simulink model "c00020M_harness"  (R2018a)
settings: Solver=ode3  StartTime=0.0  StopTime=10.0  RelTol=1e-3  EnableMultiTasking=on
undefined symbols (not defined in the file): b, DiscIntNeverNeededParam, J, K, L, PosMinimaW4, R, sigbuilder_block
(part 1 of 41)
settings Model: Creator=aarrieta  LastModifiedBy=umarkiegi
settings DataIOCC: LimitDataPoints=on  SaveFormat=Array
settings OptimizationCC: LifeSpan=inf
settings DebuggingCC: UnderspecifiedInitializationDetection=Classic  MergeDetectMultiDrivingBlocksExec=none  SolverPrmCheckMsg=warning  StateNameClashWarn=warning  SFUnexpectedBacktrackingDiag=warning  SFNoUnconditionalDefaultTransitionDiag=warning  SFExecutionAtInitializationDiag=none
settings HardwareCC: ProdBitPerPointer=32  ProdBitPerSizeT=32  ProdBitPerPtrDiffT=32  ProdLargestAtomicFloat=None  ProdIntDivRoundTo=Undefined  ProdEndianess=Unspecified  ProdWordSize=32  ProdHWDeviceType=32-bit Generic
settings ModelReferenceCC: PropagateSignalLabelsOutOfModel=off
settings CodeAppCC: StateflowObjectComments=on
settings GRTTargetCC: TargetLangStandard=C89/C90 (ANSI)  GeneratePreprocessorConditionals=Disable all
settings ConfigComp: CovMetricSettings=dw  CovHtmlReporting=on  CovSaveCumulativeToWorkspaceVar=on  CovSaveSingleToWorkspaceVar=on  CovExternalEMLEnable=off  DVMaxTestCaseSteps=20  DVTestSuiteOptimization=CombinedObjectives (Nonlinear Extended)  DVDetectFloatOverflow=off

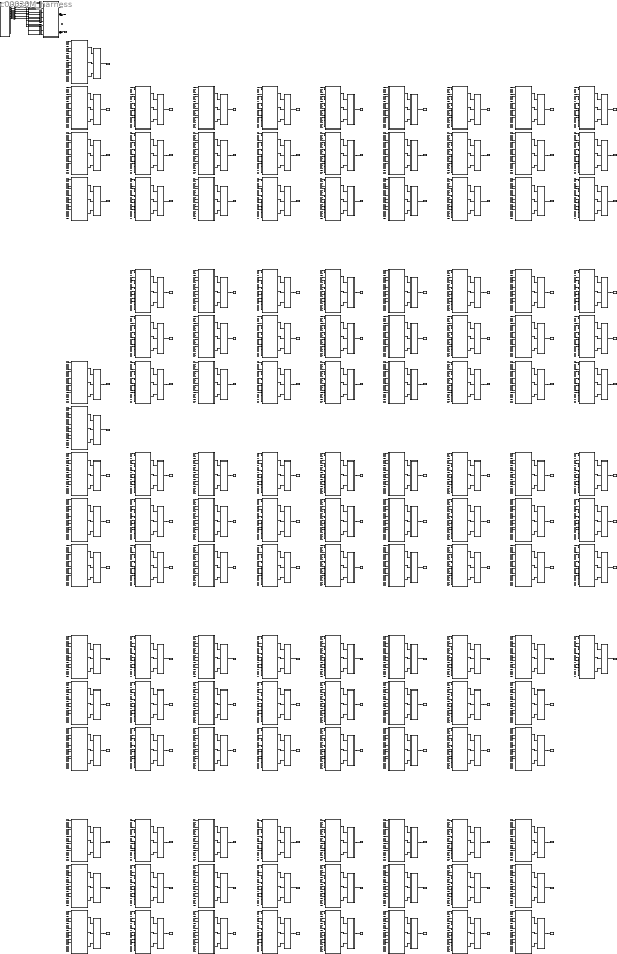
== system c00020M_harness ==
  CPSUT : Subsystem
  Eval : Subsystem
  Eval1 : Subsystem
  Eval10 : Subsystem
  Eval101 : Subsystem
  Eval102 : Subsystem
  Eval103 : Subsystem
  Eval105 : Subsystem
  Eval106 : Subsystem
  Eval107 : Subsystem
  Eval109 : Subsystem
  Eval11 : Subsystem
  Eval110 : Subsystem
  Eval111 : Subsystem
  Eval113 : Subsystem
  Eval114 : Subsystem
  Eval115 : Subsystem
  Eval117 : Subsystem
  Eval118 : Subsystem
  Eval119 : Subsystem
  Eval121 : Subsystem
  Eval122 : Subsystem
  Eval123 : Subsystem
  Eval125 : Subsystem
  Eval126 : Subsystem
  Eval127 : Subsystem
  Eval129 : Subsystem
  Eval13 : Subsystem
  Eval130 : Subsystem
  Eval131 : Subsystem
  Eval133 : Subsystem
  Eval134 : Subsystem
  Eval135 : Subsystem
  Eval137 : Subsystem
  Eval138 : Subsystem
  Eval139 : Subsystem
  Eval14 : Subsystem
  Eval141 : Subsystem
  Eval142 : Subsystem
  Eval143 : Subsystem
  Eval145 : Subsystem
  Eval146 : Subsystem
  Eval147 : Subsystem
  Eval149 : Subsystem
  Eval15 : Subsystem
  Eval150 : Subsystem
  Eval151 : Subsystem
  Eval153 : Subsystem
  Eval154 : Subsystem
  Eval155 : Subsystem
  Eval157 : Subsystem
  Eval158 : Subsystem
  Eval159 : Subsystem
  Eval161 : Subsystem
  Eval162 : Subsystem
  Eval163 : Subsystem
  Eval165 : Subsystem
  Eval166 : Subsystem
  Eval167 : Subsystem
  Eval169 : Subsystem
  Eval17 : Subsystem
  Eval170 : Subsystem
  Eval171 : Subsystem
  Eval173 : Subsystem
  Eval18 : Subsystem
  Eval19 : Subsystem
  Eval2 : Subsystem
  Eval21 : Subsystem
  Eval22 : Subsystem
  Eval23 : Subsystem
  Eval25 : Subsystem
  Eval26 : Subsystem
  Eval27 : Subsystem
  Eval29 : Subsystem
  Eval3 : Subsystem
  Eval30 : Subsystem
  Eval31 : Subsystem
  Eval33 : Subsystem
  Eval34 : Subsystem
  Eval35 : Subsystem
  Eval37 : Subsystem
  Eval38 : Subsystem
  Eval39 : Subsystem
  Eval41 : Subsystem
  Eval42 : Subsystem
  Eval43 : Subsystem
  Eval45 : Subsystem
  Eval46 : Subsystem
  Eval47 : Subsystem
  Eval49 : Subsystem
  Eval50 : Subsystem
  Eval51 : Subsystem
  Eval53 : Subsystem
  Eval54 : Subsystem
  Eval55 : Subsystem
  Eval57 : Subsystem
  Eval58 : Subsystem
  Eval59 : Subsystem
  Eval61 : Subsystem
  Eval62 : Subsystem
  Eval63 : Subsystem
  Eval65 : Subsystem
  Eval66 : Subsystem
  Eval67 : Subsystem
  Eval69 : Subsystem
  Eval7 : Subsystem
  Eval70 : Subsystem
  Eval71 : Subsystem
  Eval73 : Subsystem
  Eval74 : Subsystem
  Eval75 : Subsystem
  Eval77 : Subsystem
  Eval78 : Subsystem
  Eval79 : Subsystem
  Eval8 : Subsystem
  Eval81 : Subsystem
  Eval82 : Subsystem
  Eval83 : Subsystem
  Eval85 : Subsystem
  Eval86 : Subsystem
  Eval87 : Subsystem
  Eval89 : Subsystem
  Eval9 : Subsystem
  Eval90 : Subsystem
  Eval91 : Subsystem
  Eval93 : Subsystem
  Eval94 : Subsystem
  Eval95 : Subsystem
  Eval97 : Subsystem
  Eval98 : Subsystem
  Eval99 : Subsystem
  Inputs : Subsystem  Tag=STV Subsys  LoadFcn=sigbuilder_block('load');  StartFcn=sigbuilder_block('start');  StopFcn=sigbuilder_block('stop');  ClipboardFcn=sigbuilder_block('clipboard');  mask(Sigbuilder block){tuvar=[0:10]}
      mask init:
      | if ~strcmp(get_param(bdroot(gcb),'SimulationStatus'),'stopped'),tuvar = sigbuilder_block('maskInit'); end
      settings: CopyFcn=sigbuilder_block('copy');  DeleteFcn=sigbuilder_block('delete');  ModelCloseFcn=sigbuilder_block('modelClose');  PreSaveFcn=sigbuilder_block('preSave');  PauseFcn=sigbuilder_block('pause');  ContinueFcn=sigbuilder_block('continue');  NameChangeFcn=sigbuilder_block('namechange');  OpenFcn=sigbuilder_block('open');  CloseFcn=sigbuilder_block('close');
      mask Display: plot(0, 0, 100, 100,[2, 2, 32, 32, 2], [68, 8, 8, 68, 68],[32, 2], [38, 38], [32, 19, 2],[53, 60, 44], [32, 17, 17, 2],[16, 16, 31, 31]);txt = getActiveGroup(gcbh);text(2, 100, txt,'verticalAlignment', 'top');
  M001 : Subsystem
  M002 : Subsystem
  M003 : Subsystem
  M004 : Subsystem
  M008 : Subsystem
  M009 : Subsystem
  M010 : Subsystem
  M011 : Subsystem
  M012 : Subsystem
  M014 : Subsystem
  M015 : Subsystem
  M016 : Subsystem
  M018 : Subsystem
  M019 : Subsystem
  M020 : Subsystem
  M022 : Subsystem
  M023 : Subsystem
  M024 : Subsystem
  M026 : Subsystem
  M027 : Subsystem
  M028 : Subsystem
  M030 : Subsystem
  M031 : Subsystem
  M032 : Subsystem
  M034 : Subsystem
  M035 : Subsystem
  M036 : Subsystem
  M038 : Subsystem
  M039 : Subsystem
  M040 : Subsystem
  M042 : Subsystem
  M043 : Subsystem
  M044 : Subsystem
  M046 : Subsystem
  M047 : Subsystem
  M048 : Subsystem
  M050 : Subsystem
  M051 : Subsystem
  M052 : Subsystem
  M054 : Subsystem
  M055 : Subsystem
  M056 : Subsystem
  M058 : Subsystem
  M059 : Subsystem
  M060 : Subsystem
  M062 : Subsystem
  M063 : Subsystem
  M064 : Subsystem
  M066 : Subsystem
  M067 : Subsystem
  M068 : Subsystem
  M070 : Subsystem
  M071 : Subsystem
  M072 : Subsystem
  M074 : Subsystem
  M075 : Subsystem
  M076 : Subsystem
  M078 : Subsystem
  M079 : Subsystem
  M080 : Subsystem
  M082 : Subsystem
  M083 : Subsystem
  M084 : Subsystem
  M086 : Subsystem
  M087 : Subsystem
  M088 : Subsystem
  M090 : Subsystem
  M091 : Subsystem
  M092 : Subsystem
  M094 : Subsystem
  M095 : Subsystem
  M096 : Subsystem
  M098 : Subsystem
  M099 : Subsystem
  M100 : Subsystem
  M102 : Subsystem
  M103 : Subsystem
  M104 : Subsystem
  M106 : Subsystem
  M107 : Subsystem
  M108 : Subsystem
  M110 : Subsystem
  M111 : Subsystem
  M112 : Subsystem
  M114 : Subsystem
  M115 : Subsystem
  M116 : Subsystem
  M118 : Subsystem
  M119 : Subsystem
  M120 : Subsystem
  M122 : Subsystem
  M123 : Subsystem
  M124 : Subsystem
  M126 : Subsystem
  M127 : Subsystem
  M128 : Subsystem
  M130 : Subsystem
  M131 : Subsystem
  M132 : Subsystem
  M134 : Subsystem
  M135 : Subsystem
  M136 : Subsystem
  M138 : Subsystem
  M139 : Subsystem
  M140 : Subsystem
  M142 : Subsystem
  M143 : Subsystem
  M144 : Subsystem
  M146 : Subsystem
  M147 : Subsystem
  M148 : Subsystem
  M150 : Subsystem
  M151 : Subsystem
  M152 : Subsystem
  M154 : Subsystem
  M155 : Subsystem
  M156 : Subsystem
  M158 : Subsystem
  M159 : Subsystem
  M160 : Subsystem
  M162 : Subsystem
  M163 : Subsystem
  M164 : Subsystem
  M166 : Subsystem
  M167 : Subsystem
  M168 : Subsystem
  M170 : Subsystem
  M171 : Subsystem
  M172 : Subsystem
  M174 : Subsystem
  To Workspace : ToWorkspace  VariableName=mutant001  SampleTime=-1
  To Workspace1 : ToWorkspace  VariableName=mutant002  SampleTime=-1
  To Workspace10 : ToWorkspace  VariableName=mutant011  SampleTime=-1
  To Workspace101 : ToWorkspace  VariableName=mutant102  SampleTime=-1
  To Workspace102 : ToWorkspace  VariableName=mutant103  SampleTime=-1
  To Workspace103 : ToWorkspace  VariableName=mutant104  SampleTime=-1
  To Workspace105 : ToWorkspace  VariableName=mutant106  SampleTime=-1
  To Workspace106 : ToWorkspace  VariableName=mutant107  SampleTime=-1
  To Workspace107 : ToWorkspace  VariableName=mutant108  SampleTime=-1
  To Workspace109 : ToWorkspace  VariableName=mutant110  SampleTime=-1
  To Workspace11 : ToWorkspace  VariableName=mutant012  SampleTime=-1
  To Workspace110 : ToWorkspace  VariableName=mutant111  SampleTime=-1
  To Workspace111 : ToWorkspace  VariableName=mutant112  SampleTime=-1
  To Workspace113 : ToWorkspace  VariableName=mutant114  SampleTime=-1
  To Workspace114 : ToWorkspace  VariableName=mutant115  SampleTime=-1
  To Workspace115 : ToWorkspace  VariableName=mutant116  SampleTime=-1
  To Workspace117 : ToWorkspace  VariableName=mutant118  SampleTime=-1
  To Workspace118 : ToWorkspace  VariableName=mutant119  SampleTime=-1
  To Workspace119 : ToWorkspace  VariableName=mutant120  SampleTime=-1
  To Workspace121 : ToWorkspace  VariableName=mutant122  SampleTime=-1
  To Workspace122 : ToWorkspace  VariableName=mutant123  SampleTime=-1
  To Workspace123 : ToWorkspace  VariableName=mutant124  SampleTime=-1
  To Workspace125 : ToWorkspace  VariableName=mutant126  SampleTime=-1
  To Workspace126 : ToWorkspace  VariableName=mutant127  SampleTime=-1
  To Workspace127 : ToWorkspace  VariableName=mutant128  SampleTime=-1
  To Workspace129 : ToWorkspace  VariableName=mutant130  SampleTime=-1
  To Workspace13 : ToWorkspace  VariableName=mutant014  SampleTime=-1
  To Workspace130 : ToWorkspace  VariableName=mutant131  SampleTime=-1
  To Workspace131 : ToWorkspace  VariableName=mutant132  SampleTime=-1
  To Workspace133 : ToWorkspace  VariableName=mutant134  SampleTime=-1
  To Workspace134 : ToWorkspace  VariableName=mutant135  SampleTime=-1
  To Workspace135 : ToWorkspace  VariableName=mutant136  SampleTime=-1
  To Workspace137 : ToWorkspace  VariableName=mutant138  SampleTime=-1
  To Workspace138 : ToWorkspace  VariableName=mutant139  SampleTime=-1
  To Workspace139 : ToWorkspace  VariableName=mutant140  SampleTime=-1
  To Workspace14 : ToWorkspace  VariableName=mutant015  SampleTime=-1
  To Workspace141 : ToWorkspace  VariableName=mutant142  SampleTime=-1
  To Workspace142 : ToWorkspace  VariableName=mutant143  SampleTime=-1
  To Workspace143 : ToWorkspace  VariableName=mutant144  SampleTime=-1
  To Workspace145 : ToWorkspace  VariableName=mutant146  SampleTime=-1
  To Workspace146 : ToWorkspace  VariableName=mutant147  SampleTime=-1
  To Workspace147 : ToWorkspace  VariableName=mutant148  SampleTime=-1
  To Workspace149 : ToWorkspace  VariableName=mutant150  SampleTime=-1
  To Workspace15 : ToWorkspace  VariableName=mutant016  SampleTime=-1
  To Workspace150 : ToWorkspace  VariableName=mutant151  SampleTime=-1
  To Workspace151 : ToWorkspace  VariableName=mutant152  SampleTime=-1
  To Workspace153 : ToWorkspace  VariableName=mutant154  SampleTime=-1
  To Workspace154 : ToWorkspace  VariableName=mutant155  SampleTime=-1
  To Workspace155 : ToWorkspace  VariableName=mutant156  SampleTime=-1
  To Workspace157 : ToWorkspace  VariableName=mutant158  SampleTime=-1
  To Workspace158 : ToWorkspace  VariableName=mutant159  SampleTime=-1
  To Workspace159 : ToWorkspace  VariableName=mutant160  SampleTime=-1
  To Workspace161 : ToWorkspace  VariableName=mutant162  SampleTime=-1
  To Workspace162 : ToWorkspace  VariableName=mutant163  SampleTime=-1
  To Workspace163 : ToWorkspace  VariableName=mutant164  SampleTime=-1
  To Workspace165 : ToWorkspace  VariableName=mutant166  SampleTime=-1
  To Workspace166 : ToWorkspace  VariableName=mutant167  SampleTime=-1
  To Workspace167 : ToWorkspace  VariableName=mutant168  SampleTime=-1
  To Workspace169 : ToWorkspace  VariableName=mutant170  SampleTime=-1
  To Workspace17 : ToWorkspace  VariableName=mutant018  SampleTime=-1
  To Workspace170 : ToWorkspace  VariableName=mutant171  SampleTime=-1
  To Workspace171 : ToWorkspace  VariableName=mutant172  SampleTime=-1
  To Workspace173 : ToWorkspace  VariableName=mutant174  SampleTime=-1
  To Workspace18 : ToWorkspace  VariableName=mutant019  SampleTime=-1
  To Workspace19 : ToWorkspace  VariableName=mutant020  SampleTime=-1
  To Workspace2 : ToWorkspace  VariableName=mutant003  SampleTime=-1
  To Workspace21 : ToWorkspace  VariableName=mutant022  SampleTime=-1
  To Workspace22 : ToWorkspace  VariableName=mutant023  SampleTime=-1
  To Workspace23 : ToWorkspace  VariableName=mutant024  SampleTime=-1
  To Workspace25 : ToWorkspace  VariableName=mutant026  SampleTime=-1
  To Workspace26 : ToWorkspace  VariableName=mutant027  SampleTime=-1
  To Workspace27 : ToWorkspace  VariableName=mutant028  SampleTime=-1
  To Workspace29 : ToWorkspace  VariableName=mutant030  SampleTime=-1
  To Workspace3 : ToWorkspace  VariableName=mutant004  SampleTime=-1
  To Workspace30 : ToWorkspace  VariableName=mutant031  SampleTime=-1
  To Workspace31 : ToWorkspace  VariableName=mutant032  SampleTime=-1
  To Workspace33 : ToWorkspace  VariableName=mutant034  SampleTime=-1
  To Workspace34 : ToWorkspace  VariableName=mutant035  SampleTime=-1
  To Workspace35 : ToWorkspace  VariableName=mutant036  SampleTime=-1
  To Workspace37 : ToWorkspace  VariableName=mutant038  SampleTime=-1
  To Workspace38 : ToWorkspace  VariableName=mutant039  SampleTime=-1
  To Workspace39 : ToWorkspace  VariableName=mutant040  SampleTime=-1
  To Workspace41 : ToWorkspace  VariableName=mutant042  SampleTime=-1
  To Workspace42 : ToWorkspace  VariableName=mutant043  SampleTime=-1
  To Workspace43 : ToWorkspace  VariableName=mutant044  SampleTime=-1
  To Workspace45 : ToWorkspace  VariableName=mutant046  SampleTime=-1
  To Workspace46 : ToWorkspace  VariableName=mutant047  SampleTime=-1
  To Workspace47 : ToWorkspace  VariableName=mutant048  SampleTime=-1
  To Workspace49 : ToWorkspace  VariableName=mutant050  SampleTime=-1
  To Workspace50 : ToWorkspace  VariableName=mutant051  SampleTime=-1
  To Workspace51 : ToWorkspace  VariableName=mutant052  SampleTime=-1
  To Workspace53 : ToWorkspace  VariableName=mutant054  SampleTime=-1
  To Workspace54 : ToWorkspace  VariableName=mutant055  SampleTime=-1
  To Workspace55 : ToWorkspace  VariableName=mutant056  SampleTime=-1
  To Workspace57 : ToWorkspace  VariableName=mutant058  SampleTime=-1
  To Workspace58 : ToWorkspace  VariableName=mutant059  SampleTime=-1
  To Workspace59 : ToWorkspace  VariableName=mutant060  SampleTime=-1
  To Workspace61 : ToWorkspace  VariableName=mutant062  SampleTime=-1
  To Workspace62 : ToWorkspace  VariableName=mutant063  SampleTime=-1
  To Workspace63 : ToWorkspace  VariableName=mutant064  SampleTime=-1
  To Workspace65 : ToWorkspace  VariableName=mutant066  SampleTime=-1
  To Workspace66 : ToWorkspace  VariableName=mutant067  SampleTime=-1
  To Workspace67 : ToWorkspace  VariableName=mutant068  SampleTime=-1
  To Workspace69 : ToWorkspace  VariableName=mutant070  SampleTime=-1
  To Workspace7 : ToWorkspace  VariableName=mutant008  SampleTime=-1
  To Workspace70 : ToWorkspace  VariableName=mutant071  SampleTime=-1
  To Workspace71 : ToWorkspace  VariableName=mutant072  SampleTime=-1
  To Workspace73 : ToWorkspace  VariableName=mutant074  SampleTime=-1
  To Workspace74 : ToWorkspace  VariableName=mutant075  SampleTime=-1
  To Workspace75 : ToWorkspace  VariableName=mutant076  SampleTime=-1
  To Workspace77 : ToWorkspace  VariableName=mutant078  SampleTime=-1
  To Workspace78 : ToWorkspace  VariableName=mutant079  SampleTime=-1
  To Workspace79 : ToWorkspace  VariableName=mutant080  SampleTime=-1
  To Workspace8 : ToWorkspace  VariableName=mutant009  SampleTime=-1
  To Workspace81 : ToWorkspace  VariableName=mutant082  SampleTime=-1
  To Workspace82 : ToWorkspace  VariableName=mutant083  SampleTime=-1
  To Workspace83 : ToWorkspace  VariableName=mutant084  SampleTime=-1
  To Workspace85 : ToWorkspace  VariableName=mutant086  SampleTime=-1
  To Workspace86 : ToWorkspace  VariableName=mutant087  SampleTime=-1
  To Workspace87 : ToWorkspace  VariableName=mutant088  SampleTime=-1
  To Workspace89 : ToWorkspace  VariableName=mutant090  SampleTime=-1
  To Workspace9 : ToWorkspace  VariableName=mutant010  SampleTime=-1
  To Workspace90 : ToWorkspace  VariableName=mutant091  SampleTime=-1
  To Workspace91 : ToWorkspace  VariableName=mutant092  SampleTime=-1
  To Workspace93 : ToWorkspace  VariableName=mutant094  SampleTime=-1
  To Workspace94 : ToWorkspace  VariableName=mutant095  SampleTime=-1
  To Workspace95 : ToWorkspace  VariableName=mutant096  SampleTime=-1
  To Workspace97 : ToWorkspace  VariableName=mutant098  SampleTime=-1
  To Workspace98 : ToWorkspace  VariableName=mutant099  SampleTime=-1
  To Workspace99 : ToWorkspace  VariableName=mutant100  SampleTime=-1
  dtc_DW1 : DataTypeConversion
  dtc_DW4 : DataTypeConversion
  dtc_LD : DataTypeConversion
  dtc_O1 : DataTypeConversion
  dtc_O2 : DataTypeConversion
  dtc_O4 : DataTypeConversion
  dtc_P1W2 : DataTypeConversion
  dtc_P3W4 : DataTypeConversion
  W1Pos : Outport
  W2Pos : Outport  Port=2
  W4Pos : Outport  Port=3
  tag scope: out1=global, out2=global, out3=global, out4=global
  wires:
  CPSUT/2(W2Pos) -> [out2], W2Pos/1
  CPSUT/3(W4Pos) -> W4Pos/1, [out4]
  [in1] -> M001/1(DW1)
  [in4] -> M001/2(DW4)
  [in5] -> M001/3(P1W2)
  [in8] -> M001/4(P3W4)
  [in10] -> M001/5(O1)
  [in11] -> M001/6(O2)
  [in13] -> M001/7(O4)
  [in14] -> M001/8(LD)
  CPSUT/1(W1Pos) -> [out1], W1Pos/1
  M001/1(W1Pos) -> Eval/1(In1)
  M001/2(W2Pos) -> Eval/2(In2)
  M001/3(W4Pos) -> Eval/3(In4)
  Eval/1(Out1) -> To Workspace/1
  [in1] -> M002/1(DW1)
  [in4] -> M002/2(DW4)
  [in5] -> M002/3(P1W2)
  [in8] -> M002/4(P3W4)
  [in10] -> M002/5(O1)
  [in11] -> M002/6(O2)
  [in13] -> M002/7(O4)
  [in14] -> M002/8(LD)
  M002/1(W1Pos) -> Eval1/1(In1)
  M002/2(W2Pos) -> Eval1/2(In2)
  M002/3(W4Pos) -> Eval1/3(In4)
  Eval1/1(Out1) -> To Workspace1/1
  [in1] -> M003/1(DW1)
  [in4] -> M003/2(DW4)
  [in5] -> M003/3(P1W2)
  [in8] -> M003/4(P3W4)
  [in10] -> M003/5(O1)
  [in11] -> M003/6(O2)
  [in13] -> M003/7(O4)
  [in14] -> M003/8(LD)
  M003/1(W1Pos) -> Eval2/1(In1)
  M003/2(W2Pos) -> Eval2/2(In2)
  M003/3(W4Pos) -> Eval2/3(In4)
  Eval2/1(Out1) -> To Workspace2/1
  [in1] -> M004/1(DW1)
  [in4] -> M004/2(DW4)
  [in5] -> M004/3(P1W2)
  [in8] -> M004/4(P3W4)
  [in10] -> M004/5(O1)
  [in11] -> M004/6(O2)
  [in13] -> M004/7(O4)
  [in14] -> M004/8(LD)
  M004/1(W1Pos) -> Eval3/1(In1)
  M004/2(W2Pos) -> Eval3/2(In2)
  M004/3(W4Pos) -> Eval3/3(In4)
  Eval3/1(Out1) -> To Workspace3/1
  [in1] -> M008/1(DW1)
  [in4] -> M008/2(DW4)
  [in5] -> M008/3(P1W2)
  [in8] -> M008/4(P3W4)
  [in10] -> M008/5(O1)
  [in11] -> M008/6(O2)
  [in13] -> M008/7(O4)
  [in14] -> M008/8(LD)
  M008/1(W1Pos) -> Eval7/1(In1)
  M008/2(W2Pos) -> Eval7/2(In2)
  M008/3(W4Pos) -> Eval7/3(In4)
  Eval7/1(Out1) -> To Workspace7/1
  [in1] -> M009/1(DW1)
  [in4] -> M009/2(DW4)
  [in5] -> M009/3(P1W2)
  [in8] -> M009/4(P3W4)
  [in10] -> M009/5(O1)
  [in11] -> M009/6(O2)
  [in13] -> M009/7(O4)
  [in14] -> M009/8(LD)
  M009/1(W1Pos) -> Eval8/1(In1)
  M009/2(W2Pos) -> Eval8/2(In2)
  M009/3(W4Pos) -> Eval8/3(In4)
  Eval8/1(Out1) -> To Workspace8/1
  [in1] -> M010/1(DW1)
  [in4] -> M010/2(DW4)
  [in5] -> M010/3(P1W2)
  [in8] -> M010/4(P3W4)
  [in10] -> M010/5(O1)
  [in11] -> M010/6(O2)
  [in13] -> M010/7(O4)
  [in14] -> M010/8(LD)
  M010/1(W1Pos) -> Eval9/1(In1)
  M010/2(W2Pos) -> Eval9/2(In2)
  M010/3(W4Pos) -> Eval9/3(In4)
  Eval9/1(Out1) -> To Workspace9/1
  [in1] -> M011/1(DW1)
  [in4] -> M011/2(DW4)
  [in5] -> M011/3(P1W2)
  [in8] -> M011/4(P3W4)
  [in10] -> M011/5(O1)
  [in11] -> M011/6(O2)
  [in13] -> M011/7(O4)
  [in14] -> M011/8(LD)
  M011/1(W1Pos) -> Eval10/1(In1)
  M011/2(W2Pos) -> Eval10/2(In2)
  M011/3(W4Pos) -> Eval10/3(In4)
  Eval10/1(Out1) -> To Workspace10/1
  [in1] -> M012/1(DW1)
  [in4] -> M012/2(DW4)
  [in5] -> M012/3(P1W2)
  [in8] -> M012/4(P3W4)
  [in10] -> M012/5(O1)
  [in11] -> M012/6(O2)
  [in13] -> M012/7(O4)
  [in14] -> M012/8(LD)
  M012/1(W1Pos) -> Eval11/1(In1)
  M012/2(W2Pos) -> Eval11/2(In2)
  M012/3(W4Pos) -> Eval11/3(In4)
  Eval11/1(Out1) -> To Workspace11/1
  [in1] -> M014/1(DW1)
  [in4] -> M014/2(DW4)
  [in5] -> M014/3(P1W2)
  [in8] -> M014/4(P3W4)
  [in10] -> M014/5(O1)
  [in11] -> M014/6(O2)
  [in13] -> M014/7(O4)
  [in14] -> M014/8(LD)
  M014/1(W1Pos) -> Eval13/1(In1)
  M014/2(W2Pos) -> Eval13/2(In2)
  M014/3(W4Pos) -> Eval13/3(In4)
  Eval13/1(Out1) -> To Workspace13/1
  [in1] -> M015/1(DW1)
  [in4] -> M015/2(DW4)
  [in5] -> M015/3(P1W2)
  [in8] -> M015/4(P3W4)
  [in10] -> M015/5(O1)
  [in11] -> M015/6(O2)
  [in13] -> M015/7(O4)
  [in14] -> M015/8(LD)
  M015/1(W1Pos) -> Eval14/1(In1)
  M015/2(W2Pos) -> Eval14/2(In2)
  M015/3(W4Pos) -> Eval14/3(In4)
  Eval14/1(Out1) -> To Workspace14/1
  [in1] -> M016/1(DW1)
  [in4] -> M016/2(DW4)
  [in5] -> M016/3(P1W2)
  [in8] -> M016/4(P3W4)
  [in10] -> M016/5(O1)
  [in11] -> M016/6(O2)
  [in13] -> M016/7(O4)
  [in14] -> M016/8(LD)
  M016/1(W1Pos) -> Eval15/1(In1)
  M016/2(W2Pos) -> Eval15/2(In2)
  M016/3(W4Pos) -> Eval15/3(In4)
  Eval15/1(Out1) -> To Workspace15/1
  [in1] -> M018/1(DW1)
  [in4] -> M018/2(DW4)
  [in5] -> M018/3(P1W2)
  [in8] -> M018/4(P3W4)
  [in10] -> M018/5(O1)
  [in11] -> M018/6(O2)
  [in13] -> M018/7(O4)
  [in14] -> M018/8(LD)
  M018/1(W1Pos) -> Eval17/1(In1)
  M018/2(W2Pos) -> Eval17/2(In2)
  M018/3(W4Pos) -> Eval17/3(In4)
  Eval17/1(Out1) -> To Workspace17/1
  [in1] -> M019/1(DW1)
  [in4] -> M019/2(DW4)
  [in5] -> M019/3(P1W2)
  [in8] -> M019/4(P3W4)
  [in10] -> M019/5(O1)
  [in11] -> M019/6(O2)
  [in13] -> M019/7(O4)
  [in14] -> M019/8(LD)
  M019/1(W1Pos) -> Eval18/1(In1)
  M019/2(W2Pos) -> Eval18/2(In2)
  M019/3(W4Pos) -> Eval18/3(In4)
  Eval18/1(Out1) -> To Workspace18/1
  [in1] -> M020/1(DW1)
  [in4] -> M020/2(DW4)
  [in5] -> M020/3(P1W2)
  [in8] -> M020/4(P3W4)
  [in10] -> M020/5(O1)
  [in11] -> M020/6(O2)
  [in13] -> M020/7(O4)
  [in14] -> M020/8(LD)
  M020/1(W1Pos) -> Eval19/1(In1)
  M020/2(W2Pos) -> Eval19/2(In2)
  M020/3(W4Pos) -> Eval19/3(In4)
  Eval19/1(Out1) -> To Workspace19/1
  [in1] -> M022/1(DW1)
  [in4] -> M022/2(DW4)
  [in5] -> M022/3(P1W2)
  [in8] -> M022/4(P3W4)
  [in10] -> M022/5(O1)
  [in11] -> M022/6(O2)
  [in13] -> M022/7(O4)
  [in14] -> M022/8(LD)
  M022/1(W1Pos) -> Eval21/1(In1)
  M022/2(W2Pos) -> Eval21/2(In2)
  M022/3(W4Pos) -> Eval21/3(In4)
  Eval21/1(Out1) -> To Workspace21/1
  [in1] -> M023/1(DW1)
  [in4] -> M023/2(DW4)
  [in5] -> M023/3(P1W2)
  [in8] -> M023/4(P3W4)
  [in10] -> M023/5(O1)
  [in11] -> M023/6(O2)
  [in13] -> M023/7(O4)
  [in14] -> M023/8(LD)
  M023/1(W1Pos) -> Eval22/1(In1)
  M023/2(W2Pos) -> Eval22/2(In2)
  M023/3(W4Pos) -> Eval22/3(In4)
  Eval22/1(Out1) -> To Workspace22/1
  [in1] -> M024/1(DW1)
  [in4] -> M024/2(DW4)
  [in5] -> M024/3(P1W2)
  [in8] -> M024/4(P3W4)
  [in10] -> M024/5(O1)
  [in11] -> M024/6(O2)
  [in13] -> M024/7(O4)
  [in14] -> M024/8(LD)
  M024/1(W1Pos) -> Eval23/1(In1)
  M024/2(W2Pos) -> Eval23/2(In2)
  M024/3(W4Pos) -> Eval23/3(In4)
  Eval23/1(Out1) -> To Workspace23/1
  [in1] -> M026/1(DW1)
  [in4] -> M026/2(DW4)
  [in5] -> M026/3(P1W2)
  [in8] -> M026/4(P3W4)
  [in10] -> M026/5(O1)
  [in11] -> M026/6(O2)
  [in13] -> M026/7(O4)
  [in14] -> M026/8(LD)
  M026/1(W1Pos) -> Eval25/1(In1)
  M026/2(W2Pos) -> Eval25/2(In2)
  M026/3(W4Pos) -> Eval25/3(In4)
  Eval25/1(Out1) -> To Workspace25/1
  [in1] -> M027/1(DW1)
  [in4] -> M027/2(DW4)
  [in5] -> M027/3(P1W2)
  [in8] -> M027/4(P3W4)
  [in10] -> M027/5(O1)
  [in11] -> M027/6(O2)
  [in13] -> M027/7(O4)
  [in14] -> M027/8(LD)
  M027/1(W1Pos) -> Eval26/1(In1)
  M027/2(W2Pos) -> Eval26/2(In2)
  M027/3(W4Pos) -> Eval26/3(In4)
  Eval26/1(Out1) -> To Workspace26/1
  [in1] -> M028/1(DW1)
  [in4] -> M028/2(DW4)
  [in5] -> M028/3(P1W2)
  [in8] -> M028/4(P3W4)
  [in10] -> M028/5(O1)
  [in11] -> M028/6(O2)
  [in13] -> M028/7(O4)
  [in14] -> M028/8(LD)
  M028/1(W1Pos) -> Eval27/1(In1)
  M028/2(W2Pos) -> Eval27/2(In2)
  M028/3(W4Pos) -> Eval27/3(In4)
  Eval27/1(Out1) -> To Workspace27/1
  [in1] -> M030/1(DW1)
  [in4] -> M030/2(DW4)
  [in5] -> M030/3(P1W2)
  [in8] -> M030/4(P3W4)
  [in10] -> M030/5(O1)
  [in11] -> M030/6(O2)
  [in13] -> M030/7(O4)
  [in14] -> M030/8(LD)
  M030/1(W1Pos) -> Eval29/1(In1)
  M030/2(W2Pos) -> Eval29/2(In2)
  M030/3(W4Pos) -> Eval29/3(In4)
  Eval29/1(Out1) -> To Workspace29/1
  [in1] -> M031/1(DW1)
  [in4] -> M031/2(DW4)
  [in5] -> M031/3(P1W2)
  [in8] -> M031/4(P3W4)
  [in10] -> M031/5(O1)
  [in11] -> M031/6(O2)
  [in13] -> M031/7(O4)
  [in14] -> M031/8(LD)
  M031/1(W1Pos) -> Eval30/1(In1)
  M031/2(W2Pos) -> Eval30/2(In2)
  M031/3(W4Pos) -> Eval30/3(In4)
  Eval30/1(Out1) -> To Workspace30/1
  [in1] -> M032/1(DW1)
  [in4] -> M032/2(DW4)
  [in5] -> M032/3(P1W2)
  [in8] -> M032/4(P3W4)
  [in10] -> M032/5(O1)
  [in11] -> M032/6(O2)
  [in13] -> M032/7(O4)
  [in14] -> M032/8(LD)
  M032/1(W1Pos) -> Eval31/1(In1)
  M032/2(W2Pos) -> Eval31/2(In2)
  M032/3(W4Pos) -> Eval31/3(In4)
  Eval31/1(Out1) -> To Workspace31/1
  [in1] -> M034/1(DW1)
  [in4] -> M034/2(DW4)
  [in5] -> M034/3(P1W2)
  [in8] -> M034/4(P3W4)
  [in10] -> M034/5(O1)
  [in11] -> M034/6(O2)
  [in13] -> M034/7(O4)
  [in14] -> M034/8(LD)
  M034/1(W1Pos) -> Eval33/1(In1)
  M034/2(W2Pos) -> Eval33/2(In2)
  M034/3(W4Pos) -> Eval33/3(In4)
  Eval33/1(Out1) -> To Workspace33/1
  [in1] -> M035/1(DW1)
  [in4] -> M035/2(DW4)
  [in5] -> M035/3(P1W2)
  [in8] -> M035/4(P3W4)
  [in10] -> M035/5(O1)
  [in11] -> M035/6(O2)
  [in13] -> M035/7(O4)
  [in14] -> M035/8(LD)
  M035/1(W1Pos) -> Eval34/1(In1)
  M035/2(W2Pos) -> Eval34/2(In2)
  M035/3(W4Pos) -> Eval34/3(In4)
  Eval34/1(Out1) -> To Workspace34/1
  [in1] -> M036/1(DW1)
  [in4] -> M036/2(DW4)
  [in5] -> M036/3(P1W2)
  [in8] -> M036/4(P3W4)
  [in10] -> M036/5(O1)
  [in11] -> M036/6(O2)
  [in13] -> M036/7(O4)
  [in14] -> M036/8(LD)
  M036/1(W1Pos) -> Eval35/1(In1)
  M036/2(W2Pos) -> Eval35/2(In2)
  M036/3(W4Pos) -> Eval35/3(In4)
  Eval35/1(Out1) -> To Workspace35/1
  [in1] -> M038/1(DW1)
  [in4] -> M038/2(DW4)
  [in5] -> M038/3(P1W2)
  [in8] -> M038/4(P3W4)
  [in10] -> M038/5(O1)
  [in11] -> M038/6(O2)
  [in13] -> M038/7(O4)
  [in14] -> M038/8(LD)
  M038/1(W1Pos) -> Eval37/1(In1)
  M038/2(W2Pos) -> Eval37/2(In2)
  M038/3(W4Pos) -> Eval37/3(In4)
  Eval37/1(Out1) -> To Workspace37/1
  [in1] -> M039/1(DW1)
  [in4] -> M039/2(DW4)
  [in5] -> M039/3(P1W2)
  [in8] -> M039/4(P3W4)
  [in10] -> M039/5(O1)
  [in11] -> M039/6(O2)
  [in13] -> M039/7(O4)
  [in14] -> M039/8(LD)
  M039/1(W1Pos) -> Eval38/1(In1)
  M039/2(W2Pos) -> Eval38/2(In2)
  M039/3(W4Pos) -> Eval38/3(In4)
  Eval38/1(Out1) -> To Workspace38/1
  [in1] -> M040/1(DW1)
  [in4] -> M040/2(DW4)
  [in5] -> M040/3(P1W2)
  [in8] -> M040/4(P3W4)
  [in10] -> M040/5(O1)
  [in11] -> M040/6(O2)
  [in13] -> M040/7(O4)
  [in14] -> M040/8(LD)
  M040/1(W1Pos) -> Eval39/1(In1)
  M040/2(W2Pos) -> Eval39/2(In2)
  M040/3(W4Pos) -> Eval39/3(In4)
  Eval39/1(Out1) -> To Workspace39/1
  [in1] -> M042/1(DW1)
  [in4] -> M042/2(DW4)
  [in5] -> M042/3(P1W2)
  [in8] -> M042/4(P3W4)
  [in10] -> M042/5(O1)
  [in11] -> M042/6(O2)
  [in13] -> M042/7(O4)
  [in14] -> M042/8(LD)
  M042/1(W1Pos) -> Eval41/1(In1)
  M042/2(W2Pos) -> Eval41/2(In2)
  M042/3(W4Pos) -> Eval41/3(In4)
  Eval41/1(Out1) -> To Workspace41/1
  [in1] -> M043/1(DW1)
  [in4] -> M043/2(DW4)
  [in5] -> M043/3(P1W2)
  [in8] -> M043/4(P3W4)
  [in10] -> M043/5(O1)
  [in11] -> M043/6(O2)
  [in13] -> M043/7(O4)
  [in14] -> M043/8(LD)
  M043/1(W1Pos) -> Eval42/1(In1)
  M043/2(W2Pos) -> Eval42/2(In2)
  M043/3(W4Pos) -> Eval42/3(In4)
  Eval42/1(Out1) -> To Workspace42/1
  [in1] -> M044/1(DW1)
  [in4] -> M044/2(DW4)
  [in5] -> M044/3(P1W2)
  [in8] -> M044/4(P3W4)
  [in10] -> M044/5(O1)
  [in11] -> M044/6(O2)
  [in13] -> M044/7(O4)
  [in14] -> M044/8(LD)
  M044/1(W1Pos) -> Eval43/1(In1)
  M044/2(W2Pos) -> Eval43/2(In2)
  M044/3(W4Pos) -> Eval43/3(In4)
  Eval43/1(Out1) -> To Workspace43/1
  [in1] -> M046/1(DW1)
  [in4] -> M046/2(DW4)
  [in5] -> M046/3(P1W2)
  [in8] -> M046/4(P3W4)
  [in10] -> M046/5(O1)
  [in11] -> M046/6(O2)
  [in13] -> M046/7(O4)
  [in14] -> M046/8(LD)
  M046/1(W1Pos) -> Eval45/1(In1)
  M046/2(W2Pos) -> Eval45/2(In2)
  M046/3(W4Pos) -> Eval45/3(In4)
  Eval45/1(Out1) -> To Workspace45/1
  [in1] -> M047/1(DW1)
  [in4] -> M047/2(DW4)
  [in5] -> M047/3(P1W2)
  [in8] -> M047/4(P3W4)
  [in10] -> M047/5(O1)
  [in11] -> M047/6(O2)
  [in13] -> M047/7(O4)
  [in14] -> M047/8(LD)
  M047/1(W1Pos) -> Eval46/1(In1)
  M047/2(W2Pos) -> Eval46/2(In2)
  M047/3(W4Pos) -> Eval46/3(In4)
  Eval46/1(Out1) -> To Workspace46/1
  [in1] -> M048/1(DW1)
  [in4] -> M048/2(DW4)
  [in5] -> M048/3(P1W2)
  [in8] -> M048/4(P3W4)
  [in10] -> M048/5(O1)
  [in11] -> M048/6(O2)
  [in13] -> M048/7(O4)
  [in14] -> M048/8(LD)
  M048/1(W1Pos) -> Eval47/1(In1)
  M048/2(W2Pos) -> Eval47/2(In2)
  M048/3(W4Pos) -> Eval47/3(In4)
  Eval47/1(Out1) -> To Workspace47/1
  [in1] -> M050/1(DW1)
  [in4] -> M050/2(DW4)
  [in5] -> M050/3(P1W2)
  [in8] -> M050/4(P3W4)
  [in10] -> M050/5(O1)
  [in11] -> M050/6(O2)
  [in13] -> M050/7(O4)
  [in14] -> M050/8(LD)
  M050/1(W1Pos) -> Eval49/1(In1)
  M050/2(W2Pos) -> Eval49/2(In2)
  M050/3(W4Pos) -> Eval49/3(In4)
  Eval49/1(Out1) -> To Workspace49/1
  [in1] -> M051/1(DW1)
  [in4] -> M051/2(DW4)
  [in5] -> M051/3(P1W2)
  [in8] -> M051/4(P3W4)
  [in10] -> M051/5(O1)
  [in11] -> M051/6(O2)
  [in13] -> M051/7(O4)
  [in14] -> M051/8(LD)
  M051/1(W1Pos) -> Eval50/1(In1)
  M051/2(W2Pos) -> Eval50/2(In2)
  M051/3(W4Pos) -> Eval50/3(In4)
  Eval50/1(Out1) -> To Workspace50/1
  [in1] -> M052/1(DW1)
  [in4] -> M052/2(DW4)
  [in5] -> M052/3(P1W2)
  [in8] -> M052/4(P3W4)
  [in10] -> M052/5(O1)
  [in11] -> M052/6(O2)
  [in13] -> M052/7(O4)
  [in14] -> M052/8(LD)
  M052/1(W1Pos) -> Eval51/1(In1)
  M052/2(W2Pos) -> Eval51/2(In2)
  M052/3(W4Pos) -> Eval51/3(In4)
  Eval51/1(Out1) -> To Workspace51/1
  [in1] -> M054/1(DW1)
  [in4] -> M054/2(DW4)
  [in5] -> M054/3(P1W2)
  [in8] -> M054/4(P3W4)
  [in10] -> M054/5(O1)
  [in11] -> M054/6(O2)
  [in13] -> M054/7(O4)
  [in14] -> M054/8(LD)
  M054/1(W1Pos) -> Eval53/1(In1)
  M054/2(W2Pos) -> Eval53/2(In2)
  M054/3(W4Pos) -> Eval53/3(In4)
  Eval53/1(Out1) -> To Workspace53/1
  [in1] -> M055/1(DW1)
  [in4] -> M055/2(DW4)
  [in5] -> M055/3(P1W2)
  [in8] -> M055/4(P3W4)
  [in10] -> M055/5(O1)
  [in11] -> M055/6(O2)
  [in13] -> M055/7(O4)
  [in14] -> M055/8(LD)
  M055/1(W1Pos) -> Eval54/1(In1)
  M055/2(W2Pos) -> Eval54/2(In2)
  M055/3(W4Pos) -> Eval54/3(In4)
  Eval54/1(Out1) -> To Workspace54/1
  [in1] -> M056/1(DW1)
  [in4] -> M056/2(DW4)
  [in5] -> M056/3(P1W2)
  [in8] -> M056/4(P3W4)
  [in10] -> M056/5(O1)
  [in11] -> M056/6(O2)
  [in13] -> M056/7(O4)
  [in14] -> M056/8(LD)
  M056/1(W1Pos) -> Eval55/1(In1)
  M056/2(W2Pos) -> Eval55/2(In2)
  M056/3(W4Pos) -> Eval55/3(In4)
  Eval55/1(Out1) -> To Workspace55/1
  [in1] -> M058/1(DW1)
  [in4] -> M058/2(DW4)
  [in5] -> M058/3(P1W2)
  [in8] -> M058/4(P3W4)
  [in10] -> M058/5(O1)
  [in11] -> M058/6(O2)
  [in13] -> M058/7(O4)
  [in14] -> M058/8(LD)
  M058/1(W1Pos) -> Eval57/1(In1)
  M058/2(W2Pos) -> Eval57/2(In2)
  M058/3(W4Pos) -> Eval57/3(In4)
  Eval57/1(Out1) -> To Workspace57/1
  [in1] -> M059/1(DW1)
  [in4] -> M059/2(DW4)
  [in5] -> M059/3(P1W2)
  [in8] -> M059/4(P3W4)
  [in10] -> M059/5(O1)
  [in11] -> M059/6(O2)
  [in13] -> M059/7(O4)
  [in14] -> M059/8(LD)
  M059/1(W1Pos) -> Eval58/1(In1)
  M059/2(W2Pos) -> Eval58/2(In2)
  M059/3(W4Pos) -> Eval58/3(In4)
  Eval58/1(Out1) -> To Workspace58/1
  [in1] -> M060/1(DW1)
  [in4] -> M060/2(DW4)
  [in5] -> M060/3(P1W2)
  [in8] -> M060/4(P3W4)
  [in10] -> M060/5(O1)
  [in11] -> M060/6(O2)
  [in13] -> M060/7(O4)
  [in14] -> M060/8(LD)
  M060/1(W1Pos) -> Eval59/1(In1)
  M060/2(W2Pos) -> Eval59/2(In2)
  M060/3(W4Pos) -> Eval59/3(In4)
  Eval59/1(Out1) -> To Workspace59/1
  [in1] -> M062/1(DW1)
  [in4] -> M062/2(DW4)
  [in5] -> M062/3(P1W2)
  [in8] -> M062/4(P3W4)
  [in10] -> M062/5(O1)
  [in11] -> M062/6(O2)
  [in13] -> M062/7(O4)
  [in14] -> M062/8(LD)
  M062/1(W1Pos) -> Eval61/1(In1)
  M062/2(W2Pos) -> Eval61/2(In2)
  M062/3(W4Pos) -> Eval61/3(In4)
  Eval61/1(Out1) -> To Workspace61/1
  [in1] -> M063/1(DW1)
  [in4] -> M063/2(DW4)
  [in5] -> M063/3(P1W2)
  [in8] -> M063/4(P3W4)
  [in10] -> M063/5(O1)
  [in11] -> M063/6(O2)
  [in13] -> M063/7(O4)
  [in14] -> M063/8(LD)
  M063/1(W1Pos) -> Eval62/1(In1)
  M063/2(W2Pos) -> Eval62/2(In2)
  M063/3(W4Pos) -> Eval62/3(In4)
  Eval62/1(Out1) -> To Workspace62/1
  [in1] -> M064/1(DW1)
  [in4] -> M064/2(DW4)
  [in5] -> M064/3(P1W2)
  [in8] -> M064/4(P3W4)
  [in10] -> M064/5(O1)
  [in11] -> M064/6(O2)
  [in13] -> M064/7(O4)
  [in14] -> M064/8(LD)
  M064/1(W1Pos) -> Eval63/1(In1)
  M064/2(W2Pos) -> Eval63/2(In2)
  M064/3(W4Pos) -> Eval63/3(In4)
  Eval63/1(Out1) -> To Workspace63/1
  [in1] -> M066/1(DW1)
  [in4] -> M066/2(DW4)
  [in5] -> M066/3(P1W2)
  [in8] -> M066/4(P3W4)
  [in10] -> M066/5(O1)
  [in11] -> M066/6(O2)
  [in13] -> M066/7(O4)
  [in14] -> M066/8(LD)
  M066/1(W1Pos) -> Eval65/1(In1)
  M066/2(W2Pos) -> Eval65/2(In2)
  M066/3(W4Pos) -> Eval65/3(In4)
  Eval65/1(Out1) -> To Workspace65/1
  [in1] -> M067/1(DW1)
  [in4] -> M067/2(DW4)
  [in5] -> M067/3(P1W2)
  [in8] -> M067/4(P3W4)
  [in10] -> M067/5(O1)
  [in11] -> M067/6(O2)
  [in13] -> M067/7(O4)
  [in14] -> M067/8(LD)
  M067/1(W1Pos) -> Eval66/1(In1)
  M067/2(W2Pos) -> Eval66/2(In2)
  M067/3(W4Pos) -> Eval66/3(In4)
  Eval66/1(Out1) -> To Workspace66/1
  [in1] -> M068/1(DW1)
  [in4] -> M068/2(DW4)
  [in5] -> M068/3(P1W2)
  [in8] -> M068/4(P3W4)
  [in10] -> M068/5(O1)
  [in11] -> M068/6(O2)
  [in13] -> M068/7(O4)
  [in14] -> M068/8(LD)
  M068/1(W1Pos) -> Eval67/1(In1)
  M068/2(W2Pos) -> Eval67/2(In2)
  M068/3(W4Pos) -> Eval67/3(In4)
  Eval67/1(Out1) -> To Workspace67/1
  [in1] -> M070/1(DW1)
  [in4] -> M070/2(DW4)
  [in5] -> M070/3(P1W2)
  [in8] -> M070/4(P3W4)
  [in10] -> M070/5(O1)
  [in11] -> M070/6(O2)
  [in13] -> M070/7(O4)
  [in14] -> M070/8(LD)
  M070/1(W1Pos) -> Eval69/1(In1)
  M070/2(W2Pos) -> Eval69/2(In2)
  M070/3(W4Pos) -> Eval69/3(In4)
  Eval69/1(Out1) -> To Workspace69/1
  [in1] -> M071/1(DW1)
  [in4] -> M071/2(DW4)
  [in5] -> M071/3(P1W2)
  [in8] -> M071/4(P3W4)
  [in10] -> M071/5(O1)
  [in11] -> M071/6(O2)
  [in13] -> M071/7(O4)
  [in14] -> M071/8(LD)
  M071/1(W1Pos) -> Eval70/1(In1)
  M071/2(W2Pos) -> Eval70/2(In2)
  M071/3(W4Pos) -> Eval70/3(In4)
  Eval70/1(Out1) -> To Workspace70/1
  [in1] -> M072/1(DW1)
  [in4] -> M072/2(DW4)
  [in5] -> M072/3(P1W2)
  [in8] -> M072/4(P3W4)
  [in10] -> M072/5(O1)
  [in11] -> M072/6(O2)
  [in13] -> M072/7(O4)
  [in14] -> M072/8(LD)
  M072/1(W1Pos) -> Eval71/1(In1)
  M072/2(W2Pos) -> Eval71/2(In2)
  M072/3(W4Pos) -> Eval71/3(In4)
  Eval71/1(Out1) -> To Workspace71/1
  [in1] -> M074/1(DW1)
  [in4] -> M074/2(DW4)
  [in5] -> M074/3(P1W2)
  [in8] -> M074/4(P3W4)
  [in10] -> M074/5(O1)
  [in11] -> M074/6(O2)
  [in13] -> M074/7(O4)
  [in14] -> M074/8(LD)
  M074/1(W1Pos) -> Eval73/1(In1)
  M074/2(W2Pos) -> Eval73/2(In2)
  M074/3(W4Pos) -> Eval73/3(In4)
  Eval73/1(Out1) -> To Workspace73/1
  [in1] -> M075/1(DW1)
  [in4] -> M075/2(DW4)
  [in5] -> M075/3(P1W2)
  [in8] -> M075/4(P3W4)
  [in10] -> M075/5(O1)
  [in11] -> M075/6(O2)
  [in13] -> M075/7(O4)
  [in14] -> M075/8(LD)
  M075/1(W1Pos) -> Eval74/1(In1)
  M075/2(W2Pos) -> Eval74/2(In2)
  M075/3(W4Pos) -> Eval74/3(In4)
  Eval74/1(Out1) -> To Workspace74/1
  [in1] -> M076/1(DW1)
  [in4] -> M076/2(DW4)
  [in5] -> M076/3(P1W2)
  [in8] -> M076/4(P3W4)
  [in10] -> M076/5(O1)
  [in11] -> M076/6(O2)
  [in13] -> M076/7(O4)
  [in14] -> M076/8(LD)
  M076/1(W1Pos) -> Eval75/1(In1)
  M076/2(W2Pos) -> Eval75/2(In2)
  M076/3(W4Pos) -> Eval75/3(In4)
  Eval75/1(Out1) -> To Workspace75/1
  [in1] -> M078/1(DW1)
  [in4] -> M078/2(DW4)
  [in5] -> M078/3(P1W2)
  [in8] -> M078/4(P3W4)
  [in10] -> M078/5(O1)
  [in11] -> M078/6(O2)
  [in13] -> M078/7(O4)
  [in14] -> M078/8(LD)
  M078/1(W1Pos) -> Eval77/1(In1)
  M078/2(W2Pos) -> Eval77/2(In2)
  M078/3(W4Pos) -> Eval77/3(In4)
  Eval77/1(Out1) -> To Workspace77/1
  [in1] -> M079/1(DW1)
  [in4] -> M079/2(DW4)
  [in5] -> M079/3(P1W2)
  [in8] -> M079/4(P3W4)
  [in10] -> M079/5(O1)
  [in11] -> M079/6(O2)
  [in13] -> M079/7(O4)
  [in14] -> M079/8(LD)
  M079/1(W1Pos) -> Eval78/1(In1)
  M079/2(W2Pos) -> Eval78/2(In2)
  M079/3(W4Pos) -> Eval78/3(In4)
  Eval78/1(Out1) -> To Workspace78/1
  [in1] -> M080/1(DW1)
  [in4] -> M080/2(DW4)
  [in5] -> M080/3(P1W2)
  [in8] -> M080/4(P3W4)
  [in10] -> M080/5(O1)
  [in11] -> M080/6(O2)
  [in13] -> M080/7(O4)
  [in14] -> M080/8(LD)
  M080/1(W1Pos) -> Eval79/1(In1)
  M080/2(W2Pos) -> Eval79/2(In2)
  M080/3(W4Pos) -> Eval79/3(In4)
  Eval79/1(Out1) -> To Workspace79/1
  [in1] -> M082/1(DW1)
  [in4] -> M082/2(DW4)
  [in5] -> M082/3(P1W2)
  [in8] -> M082/4(P3W4)
  [in10] -> M082/5(O1)
  [in11] -> M082/6(O2)
  [in13] -> M082/7(O4)
  [in14] -> M082/8(LD)
  M082/1(W1Pos) -> Eval81/1(In1)
  M082/2(W2Pos) -> Eval81/2(In2)
  M082/3(W4Pos) -> Eval81/3(In4)
  Eval81/1(Out1) -> To Workspace81/1
  [in1] -> M083/1(DW1)
  [in4] -> M083/2(DW4)
  [in5] -> M083/3(P1W2)
  [in8] -> M083/4(P3W4)
  [in10] -> M083/5(O1)
  [in11] -> M083/6(O2)
  [in13] -> M083/7(O4)
  [in14] -> M083/8(LD)
  M083/1(W1Pos) -> Eval82/1(In1)
  M083/2(W2Pos) -> Eval82/2(In2)
  M083/3(W4Pos) -> Eval82/3(In4)
  Eval82/1(Out1) -> To Workspace82/1
  [in1] -> M084/1(DW1)
  [in4] -> M084/2(DW4)
  [in5] -> M084/3(P1W2)
  [in8] -> M084/4(P3W4)
  [in10] -> M084/5(O1)
  [in11] -> M084/6(O2)
  [in13] -> M084/7(O4)
  [in14] -> M084/8(LD)
  M084/1(W1Pos) -> Eval83/1(In1)
  M084/2(W2Pos) -> Eval83/2(In2)
  M084/3(W4Pos) -> Eval83/3(In4)
  Eval83/1(Out1) -> To Workspace83/1
  [in1] -> M086/1(DW1)
  [in4] -> M086/2(DW4)
  [in5] -> M086/3(P1W2)
  [in8] -> M086/4(P3W4)
  [in10] -> M086/5(O1)
  [in11] -> M086/6(O2)
  [in13] -> M086/7(O4)
  [in14] -> M086/8(LD)
  M086/1(W1Pos) -> Eval85/1(In1)
  M086/2(W2Pos) -> Eval85/2(In2)
  M086/3(W4Pos) -> Eval85/3(In4)
  Eval85/1(Out1) -> To Workspace85/1
  [in1] -> M087/1(DW1)
  [in4] -> M087/2(DW4)
  [in5] -> M087/3(P1W2)
  [in8] -> M087/4(P3W4)
  [in10] -> M087/5(O1)
  [in11] -> M087/6(O2)
  [in13] -> M087/7(O4)
  [in14] -> M087/8(LD)
  M087/1(W1Pos) -> Eval86/1(In1)
  M087/2(W2Pos) -> Eval86/2(In2)
  M087/3(W4Pos) -> Eval86/3(In4)
  Eval86/1(Out1) -> To Workspace86/1
  [in1] -> M088/1(DW1)
  [in4] -> M088/2(DW4)
  [in5] -> M088/3(P1W2)
  [in8] -> M088/4(P3W4)
  [in10] -> M088/5(O1)
  [in11] -> M088/6(O2)
  [in13] -> M088/7(O4)
  [in14] -> M088/8(LD)
  M088/1(W1Pos) -> Eval87/1(In1)
  M088/2(W2Pos) -> Eval87/2(In2)
  M088/3(W4Pos) -> Eval87/3(In4)
  Eval87/1(Out1) -> To Workspace87/1
  [in1] -> M090/1(DW1)
  [in4] -> M090/2(DW4)
  [in5] -> M090/3(P1W2)
  [in8] -> M090/4(P3W4)
  [in10] -> M090/5(O1)
  [in11] -> M090/6(O2)
  [in13] -> M090/7(O4)
  [in14] -> M090/8(LD)
  M090/1(W1Pos) -> Eval89/1(In1)
  M090/2(W2Pos) -> Eval89/2(In2)
  M090/3(W4Pos) -> Eval89/3(In4)
  Eval89/1(Out1) -> To Workspace89/1
  [in1] -> M091/1(DW1)
  [in4] -> M091/2(DW4)
  [in5] -> M091/3(P1W2)
  [in8] -> M091/4(P3W4)
  [in10] -> M091/5(O1)
  [in11] -> M091/6(O2)
  [in13] -> M091/7(O4)
  [in14] -> M091/8(LD)
  M091/1(W1Pos) -> Eval90/1(In1)
  M091/2(W2Pos) -> Eval90/2(In2)
  M091/3(W4Pos) -> Eval90/3(In4)
  Eval90/1(Out1) -> To Workspace90/1
  [in1] -> M092/1(DW1)
  [in4] -> M092/2(DW4)
  [in5] -> M092/3(P1W2)
  [in8] -> M092/4(P3W4)
  [in10] -> M092/5(O1)
  [in11] -> M092/6(O2)
  [in13] -> M092/7(O4)
  [in14] -> M092/8(LD)
  M092/1(W1Pos) -> Eval91/1(In1)
  M092/2(W2Pos) -> Eval91/2(In2)
  M092/3(W4Pos) -> Eval91/3(In4)
  Eval91/1(Out1) -> To Workspace91/1
  [in1] -> M094/1(DW1)
  [in4] -> M094/2(DW4)
  [in5] -> M094/3(P1W2)
  [in8] -> M094/4(P3W4)
  [in10] -> M094/5(O1)
  [in11] -> M094/6(O2)
  [in13] -> M094/7(O4)
  [in14] -> M094/8(LD)
  M094/1(W1Pos) -> Eval93/1(In1)
  M094/2(W2Pos) -> Eval93/2(In2)
  M094/3(W4Pos) -> Eval93/3(In4)
  Eval93/1(Out1) -> To Workspace93/1
  [in1] -> M095/1(DW1)
  [in4] -> M095/2(DW4)
  [in5] -> M095/3(P1W2)
  [in8] -> M095/4(P3W4)
  [in10] -> M095/5(O1)
  [in11] -> M095/6(O2)
  [in13] -> M095/7(O4)
  [in14] -> M095/8(LD)
  M095/1(W1Pos) -> Eval94/1(In1)
  M095/2(W2Pos) -> Eval94/2(In2)
  M095/3(W4Pos) -> Eval94/3(In4)
  Eval94/1(Out1) -> To Workspace94/1
  [in1] -> M096/1(DW1)
  [in4] -> M096/2(DW4)
  [in5] -> M096/3(P1W2)
  [in8] -> M096/4(P3W4)
  [in10] -> M096/5(O1)
  [in11] -> M096/6(O2)
  [in13] -> M096/7(O4)
  [in14] -> M096/8(LD)
  M096/1(W1Pos) -> Eval95/1(In1)
  M096/2(W2Pos) -> Eval95/2(In2)
  M096/3(W4Pos) -> Eval95/3(In4)
  Eval95/1(Out1) -> To Workspace95/1
  [in1] -> M098/1(DW1)
  [in4] -> M098/2(DW4)
  [in5] -> M098/3(P1W2)
  [in8] -> M098/4(P3W4)
  [in10] -> M098/5(O1)
  [in11] -> M098/6(O2)
  [in13] -> M098/7(O4)
  [in14] -> M098/8(LD)
  M098/1(W1Pos) -> Eval97/1(In1)
  M098/2(W2Pos) -> Eval97/2(In2)
  M098/3(W4Pos) -> Eval97/3(In4)
  Eval97/1(Out1) -> To Workspace97/1
  [in1] -> M099/1(DW1)
  [in4] -> M099/2(DW4)
  [in5] -> M099/3(P1W2)
  [in8] -> M099/4(P3W4)
  [in10] -> M099/5(O1)
  [in11] -> M099/6(O2)
  [in13] -> M099/7(O4)
  [in14] -> M099/8(LD)
  M099/1(W1Pos) -> Eval98/1(In1)
  M099/2(W2Pos) -> Eval98/2(In2)
  M099/3(W4Pos) -> Eval98/3(In4)
  Eval98/1(Out1) -> To Workspace98/1
  [in1] -> M100/1(DW1)
  [in4] -> M100/2(DW4)
  [in5] -> M100/3(P1W2)
  [in8] -> M100/4(P3W4)
  [in10] -> M100/5(O1)
  [in11] -> M100/6(O2)
  [in13] -> M100/7(O4)
  [in14] -> M100/8(LD)
  M100/1(W1Pos) -> Eval99/1(In1)
  M100/2(W2Pos) -> Eval99/2(In2)
  M100/3(W4Pos) -> Eval99/3(In4)
  Eval99/1(Out1) -> To Workspace99/1
  [in1] -> M102/1(DW1)
  [in4] -> M102/2(DW4)
  [in5] -> M102/3(P1W2)
  [in8] -> M102/4(P3W4)
  [in10] -> M102/5(O1)
  [in11] -> M102/6(O2)
  [in13] -> M102/7(O4)
  [in14] -> M102/8(LD)
  M102/1(W1Pos) -> Eval101/1(In1)
  M102/2(W2Pos) -> Eval101/2(In2)
  M102/3(W4Pos) -> Eval101/3(In4)
  Eval101/1(Out1) -> To Workspace101/1
  [in1] -> M103/1(DW1)
  [in4] -> M103/2(DW4)
  [in5] -> M103/3(P1W2)
  [in8] -> M103/4(P3W4)
  [in10] -> M103/5(O1)
  [in11] -> M103/6(O2)
  [in13] -> M103/7(O4)
  [in14] -> M103/8(LD)
  M103/1(W1Pos) -> Eval102/1(In1)
  M103/2(W2Pos) -> Eval102/2(In2)
  M103/3(W4Pos) -> Eval102/3(In4)
  Eval102/1(Out1) -> To Workspace102/1
  [in1] -> M104/1(DW1)
  [in4] -> M104/2(DW4)
  [in5] -> M104/3(P1W2)
  [in8] -> M104/4(P3W4)
  [in10] -> M104/5(O1)
  [in11] -> M104/6(O2)
  [in13] -> M104/7(O4)
  [in14] -> M104/8(LD)
  M104/1(W1Pos) -> Eval103/1(In1)
  M104/2(W2Pos) -> Eval103/2(In2)
  M104/3(W4Pos) -> Eval103/3(In4)
  Eval103/1(Out1) -> To Workspace103/1
  [in1] -> M106/1(DW1)
  [in4] -> M106/2(DW4)
  [in5] -> M106/3(P1W2)
  [in8] -> M106/4(P3W4)
  [in10] -> M106/5(O1)
  [in11] -> M106/6(O2)
  [in13] -> M106/7(O4)
  [in14] -> M106/8(LD)
  M106/1(W1Pos) -> Eval105/1(In1)
  M106/2(W2Pos) -> Eval105/2(In2)
  M106/3(W4Pos) -> Eval105/3(In4)
  Eval105/1(Out1) -> To Workspace105/1
  [in1] -> M107/1(DW1)
  [in4] -> M107/2(DW4)
  [in5] -> M107/3(P1W2)
  [in8] -> M107/4(P3W4)
  [in10] -> M107/5(O1)
  [in11] -> M107/6(O2)
  [in13] -> M107/7(O4)
  [in14] -> M107/8(LD)
  M107/1(W1Pos) -> Eval106/1(In1)
  M107/2(W2Pos) -> Eval106/2(In2)
  M107/3(W4Pos) -> Eval106/3(In4)
  Eval106/1(Out1) -> To Workspace106/1
  [in1] -> M108/1(DW1)
  [in4] -> M108/2(DW4)
  [in5] -> M108/3(P1W2)
  [in8] -> M108/4(P3W4)
  [in10] -> M108/5(O1)
  [in11] -> M108/6(O2)
  [in13] -> M108/7(O4)
  [in14] -> M108/8(LD)
  M108/1(W1Pos) -> Eval107/1(In1)
  M108/2(W2Pos) -> Eval107/2(In2)
  M108/3(W4Pos) -> Eval107/3(In4)
  Eval107/1(Out1) -> To Workspace107/1
  [in1] -> M110/1(DW1)
  [in4] -> M110/2(DW4)
  [in5] -> M110/3(P1W2)
  [in8] -> M110/4(P3W4)
  [in10] -> M110/5(O1)
  [in11] -> M110/6(O2)
  [in13] -> M110/7(O4)
  [in14] -> M110/8(LD)
  M110/1(W1Pos) -> Eval109/1(In1)
  M110/2(W2Pos) -> Eval109/2(In2)
  M110/3(W4Pos) -> Eval109/3(In4)
  Eval109/1(Out1) -> To Workspace109/1
  [in1] -> M111/1(DW1)
  [in4] -> M111/2(DW4)
  [in5] -> M111/3(P1W2)
  [in8] -> M111/4(P3W4)
  [in10] -> M111/5(O1)
  [in11] -> M111/6(O2)
  [in13] -> M111/7(O4)
  [in14] -> M111/8(LD)
  M111/1(W1Pos) -> Eval110/1(In1)
  M111/2(W2Pos) -> Eval110/2(In2)
  M111/3(W4Pos) -> Eval110/3(In4)
  Eval110/1(Out1) -> To Workspace110/1
  [in1] -> M112/1(DW1)
  [in4] -> M112/2(DW4)
  [in5] -> M112/3(P1W2)
  [in8] -> M112/4(P3W4)
  [in10] -> M112/5(O1)
  [in11] -> M112/6(O2)
  [in13] -> M112/7(O4)
  [in14] -> M112/8(LD)
  M112/1(W1Pos) -> Eval111/1(In1)
  M112/2(W2Pos) -> Eval111/2(In2)
  M112/3(W4Pos) -> Eval111/3(In4)
  Eval111/1(Out1) -> To Workspace111/1
  [in1] -> M114/1(DW1)
  [in4] -> M114/2(DW4)
  [in5] -> M114/3(P1W2)
  [in8] -> M114/4(P3W4)
  [in10] -> M114/5(O1)
  [in11] -> M114/6(O2)
  [in13] -> M114/7(O4)
  [in14] -> M114/8(LD)
  M114/1(W1Pos) -> Eval113/1(In1)
  M114/2(W2Pos) -> Eval113/2(In2)
  M114/3(W4Pos) -> Eval113/3(In4)
  Eval113/1(Out1) -> To Workspace113/1
  [in1] -> M115/1(DW1)
  [in4] -> M115/2(DW4)
  [in5] -> M115/3(P1W2)
  [in8] -> M115/4(P3W4)
  [in10] -> M115/5(O1)
  [in11] -> M115/6(O2)
  [in13] -> M115/7(O4)
  [in14] -> M115/8(LD)
  M115/1(W1Pos) -> Eval114/1(In1)
  M115/2(W2Pos) -> Eval114/2(In2)
  M115/3(W4Pos) -> Eval114/3(In4)
  Eval114/1(Out1) -> To Workspace114/1
  [in1] -> M116/1(DW1)
  [in4] -> M116/2(DW4)
  [in5] -> M116/3(P1W2)
  [in8] -> M116/4(P3W4)
  [in10] -> M116/5(O1)
  [in11] -> M116/6(O2)
  [in13] -> M116/7(O4)
  [in14] -> M116/8(LD)
  M116/1(W1Pos) -> Eval115/1(In1)
  M116/2(W2Pos) -> Eval115/2(In2)
  M116/3(W4Pos) -> Eval115/3(In4)
  Eval115/1(Out1) -> To Workspace115/1
  [in1] -> M118/1(DW1)
  [in4] -> M118/2(DW4)
  [in5] -> M118/3(P1W2)
  [in8] -> M118/4(P3W4)
  [in10] -> M118/5(O1)
  [in11] -> M118/6(O2)
  [in13] -> M118/7(O4)
  [in14] -> M118/8(LD)
  M118/1(W1Pos) -> Eval117/1(In1)
  M118/2(W2Pos) -> Eval117/2(In2)
  M118/3(W4Pos) -> Eval117/3(In4)
  Eval117/1(Out1) -> To Workspace117/1
  [in1] -> M119/1(DW1)
  [in4] -> M119/2(DW4)
  [in5] -> M119/3(P1W2)
  [in8] -> M119/4(P3W4)
  [in10] -> M119/5(O1)
  [in11] -> M119/6(O2)
  [in13] -> M119/7(O4)
  [in14] -> M119/8(LD)
  M119/1(W1Pos) -> Eval118/1(In1)
  M119/2(W2Pos) -> Eval118/2(In2)
  M119/3(W4Pos) -> Eval118/3(In4)
  Eval118/1(Out1) -> To Workspace118/1
  [in1] -> M120/1(DW1)
  [in4] -> M120/2(DW4)
  [in5] -> M120/3(P1W2)
  [in8] -> M120/4(P3W4)
  [in10] -> M120/5(O1)
  [in11] -> M120/6(O2)
  [in13] -> M120/7(O4)
  [in14] -> M120/8(LD)
  M120/1(W1Pos) -> Eval119/1(In1)
  M120/2(W2Pos) -> Eval119/2(In2)
  M120/3(W4Pos) -> Eval119/3(In4)
  Eval119/1(Out1) -> To Workspace119/1
  [in1] -> M122/1(DW1)
  [in4] -> M122/2(DW4)
  [in5] -> M122/3(P1W2)
  [in8] -> M122/4(P3W4)
  [in10] -> M122/5(O1)
  [in11] -> M122/6(O2)
  [in13] -> M122/7(O4)
  [in14] -> M122/8(LD)
  M122/1(W1Pos) -> Eval121/1(In1)
  M122/2(W2Pos) -> Eval121/2(In2)
  M122/3(W4Pos) -> Eval121/3(In4)
  Eval121/1(Out1) -> To Workspace121/1
  [in1] -> M123/1(DW1)
  [in4] -> M123/2(DW4)
  [in5] -> M123/3(P1W2)
  [in8] -> M123/4(P3W4)
  [in10] -> M123/5(O1)
  [in11] -> M123/6(O2)
  [in13] -> M123/7(O4)
  [in14] -> M123/8(LD)
  M123/1(W1Pos) -> Eval122/1(In1)
  M123/2(W2Pos) -> Eval122/2(In2)
  M123/3(W4Pos) -> Eval122/3(In4)
  Eval122/1(Out1) -> To Workspace122/1
  [in1] -> M124/1(DW1)
  [in4] -> M124/2(DW4)
  [in5] -> M124/3(P1W2)
  [in8] -> M124/4(P3W4)
  [in10] -> M124/5(O1)
  [in11] -> M124/6(O2)
  [in13] -> M124/7(O4)
  [in14] -> M124/8(LD)
  M124/1(W1Pos) -> Eval123/1(In1)
  M124/2(W2Pos) -> Eval123/2(In2)
  M124/3(W4Pos) -> Eval123/3(In4)
  Eval123/1(Out1) -> To Workspace123/1
  [in1] -> M126/1(DW1)
  [in4] -> M126/2(DW4)
  [in5] -> M126/3(P1W2)
  [in8] -> M126/4(P3W4)
  [in10] -> M126/5(O1)
  [in11] -> M126/6(O2)
  [in13] -> M126/7(O4)
  [in14] -> M126/8(LD)
  M126/1(W1Pos) -> Eval125/1(In1)
  M126/2(W2Pos) -> Eval125/2(In2)
  M126/3(W4Pos) -> Eval125/3(In4)
  Eval125/1(Out1) -> To Workspace125/1
  [in1] -> M127/1(DW1)
  [in4] -> M127/2(DW4)
  [in5] -> M127/3(P1W2)
  [in8] -> M127/4(P3W4)
  [in10] -> M127/5(O1)
  [in11] -> M127/6(O2)
  [in13] -> M127/7(O4)
  [in14] -> M127/8(LD)
  M127/1(W1Pos) -> Eval126/1(In1)
  M127/2(W2Pos) -> Eval126/2(In2)
  M127/3(W4Pos) -> Eval126/3(In4)
  Eval126/1(Out1) -> To Workspace126/1
  [in1] -> M128/1(DW1)
  [in4] -> M128/2(DW4)
  [in5] -> M128/3(P1W2)
  [in8] -> M128/4(P3W4)
  [in10] -> M128/5(O1)
  [in11] -> M128/6(O2)
  [in13] -> M128/7(O4)
  [in14] -> M128/8(LD)
  M128/1(W1Pos) -> Eval127/1(In1)
  M128/2(W2Pos) -> Eval127/2(In2)
  M128/3(W4Pos) -> Eval127/3(In4)
  Eval127/1(Out1) -> To Workspace127/1
  [in1] -> M130/1(DW1)
  [in4] -> M130/2(DW4)
  [in5] -> M130/3(P1W2)
  [in8] -> M130/4(P3W4)
  [in10] -> M130/5(O1)
  [in11] -> M130/6(O2)
  [in13] -> M130/7(O4)
  [in14] -> M130/8(LD)
  M130/1(W1Pos) -> Eval129/1(In1)
  M130/2(W2Pos) -> Eval129/2(In2)
  M130/3(W4Pos) -> Eval129/3(In4)
  Eval129/1(Out1) -> To Workspace129/1
  [in1] -> M131/1(DW1)
  [in4] -> M131/2(DW4)
  [in5] -> M131/3(P1W2)
  [in8] -> M131/4(P3W4)
  [in10] -> M131/5(O1)
  [in11] -> M131/6(O2)
  [in13] -> M131/7(O4)
  [in14] -> M131/8(LD)
  M131/1(W1Pos) -> Eval130/1(In1)
  M131/2(W2Pos) -> Eval130/2(In2)
  M131/3(W4Pos) -> Eval130/3(In4)
  Eval130/1(Out1) -> To Workspace130/1
  [in1] -> M132/1(DW1)
  [in4] -> M132/2(DW4)
  [in5] -> M132/3(P1W2)
  [in8] -> M132/4(P3W4)
  [in10] -> M132/5(O1)
  [in11] -> M132/6(O2)
  [in13] -> M132/7(O4)
  [in14] -> M132/8(LD)
  M132/1(W1Pos) -> Eval131/1(In1)
  M132/2(W2Pos) -> Eval131/2(In2)
  M132/3(W4Pos) -> Eval131/3(In4)
  Eval131/1(Out1) -> To Workspace131/1
  [in1] -> M134/1(DW1)
  [in4] -> M134/2(DW4)
  [in5] -> M134/3(P1W2)
  [in8] -> M134/4(P3W4)
  [in10] -> M134/5(O1)
  [in11] -> M134/6(O2)
  [in13] -> M134/7(O4)
  [in14] -> M134/8(LD)
  M134/1(W1Pos) -> Eval133/1(In1)
  M134/2(W2Pos) -> Eval133/2(In2)
  M134/3(W4Pos) -> Eval133/3(In4)
  Eval133/1(Out1) -> To Workspace133/1
  [in1] -> M135/1(DW1)
  [in4] -> M135/2(DW4)
  [in5] -> M135/3(P1W2)
  [in8] -> M135/4(P3W4)
  [in10] -> M135/5(O1)
  [in11] -> M135/6(O2)
  [in13] -> M135/7(O4)
  [in14] -> M135/8(LD)
  M135/1(W1Pos) -> Eval134/1(In1)
  M135/2(W2Pos) -> Eval134/2(In2)
  M135/3(W4Pos) -> Eval134/3(In4)
  Eval134/1(Out1) -> To Workspace134/1
  [in1] -> M136/1(DW1)
  [in4] -> M136/2(DW4)
  [in5] -> M136/3(P1W2)
  [in8] -> M136/4(P3W4)
  [in10] -> M136/5(O1)
  [in11] -> M136/6(O2)
  [in13] -> M136/7(O4)
  [in14] -> M136/8(LD)
  M136/1(W1Pos) -> Eval135/1(In1)
  M136/2(W2Pos) -> Eval135/2(In2)
  M136/3(W4Pos) -> Eval135/3(In4)
  Eval135/1(Out1) -> To Workspace135/1
  [in1] -> M138/1(DW1)
  [in4] -> M138/2(DW4)
  [in5] -> M138/3(P1W2)
  [in8] -> M138/4(P3W4)
  [in10] -> M138/5(O1)
  [in11] -> M138/6(O2)
  [in13] -> M138/7(O4)
  [in14] -> M138/8(LD)
  M138/1(W1Pos) -> Eval137/1(In1)
  M138/2(W2Pos) -> Eval137/2(In2)
  M138/3(W4Pos) -> Eval137/3(In4)
  Eval137/1(Out1) -> To Workspace137/1
  [in1] -> M139/1(DW1)
  [in4] -> M139/2(DW4)
  [in5] -> M139/3(P1W2)
  [in8] -> M139/4(P3W4)
  [in10] -> M139/5(O1)
  [in11] -> M139/6(O2)
  [in13] -> M139/7(O4)
  [in14] -> M139/8(LD)
  M139/1(W1Pos) -> Eval138/1(In1)
  M139/2(W2Pos) -> Eval138/2(In2)
  M139/3(W4Pos) -> Eval138/3(In4)
  Eval138/1(Out1) -> To Workspace138/1
  [in1] -> M140/1(DW1)
  [in4] -> M140/2(DW4)
  [in5] -> M140/3(P1W2)
  [in8] -> M140/4(P3W4)
  [in10] -> M140/5(O1)
  [in11] -> M140/6(O2)
  [in13] -> M140/7(O4)
  [in14] -> M140/8(LD)
  M140/1(W1Pos) -> Eval139/1(In1)
  M140/2(W2Pos) -> Eval139/2(In2)
  M140/3(W4Pos) -> Eval139/3(In4)
  Eval139/1(Out1) -> To Workspace139/1
  [in1] -> M142/1(DW1)
  [in4] -> M142/2(DW4)
  [in5] -> M142/3(P1W2)
  [in8] -> M142/4(P3W4)
  [in10] -> M142/5(O1)
  [in11] -> M142/6(O2)
  [in13] -> M142/7(O4)
  [in14] -> M142/8(LD)
  M142/1(W1Pos) -> Eval141/1(In1)
  M142/2(W2Pos) -> Eval141/2(In2)
  M142/3(W4Pos) -> Eval141/3(In4)
  Eval141/1(Out1) -> To Workspace141/1
  [in1] -> M143/1(DW1)
  [in4] -> M143/2(DW4)
  [in5] -> M143/3(P1W2)
  [in8] -> M143/4(P3W4)
  [in10] -> M143/5(O1)
  [in11] -> M143/6(O2)
  [in13] -> M143/7(O4)
  [in14] -> M143/8(LD)
  M143/1(W1Pos) -> Eval142/1(In1)
  M143/2(W2Pos) -> Eval142/2(In2)
  M143/3(W4Pos) -> Eval142/3(In4)
  Eval142/1(Out1) -> To Workspace142/1
  [in1] -> M144/1(DW1)
  [in4] -> M144/2(DW4)
  [in5] -> M144/3(P1W2)
  [in8] -> M144/4(P3W4)
  [in10] -> M144/5(O1)
  [in11] -> M144/6(O2)
  [in13] -> M144/7(O4)
  [in14] -> M144/8(LD)
  M144/1(W1Pos) -> Eval143/1(In1)
  M144/2(W2Pos) -> Eval143/2(In2)
  M144/3(W4Pos) -> Eval143/3(In4)
  Eval143/1(Out1) -> To Workspace143/1
  [in1] -> M146/1(DW1)
  [in4] -> M146/2(DW4)
  [in5] -> M146/3(P1W2)
  [in8] -> M146/4(P3W4)
  [in10] -> M146/5(O1)
  [in11] -> M146/6(O2)
  [in13] -> M146/7(O4)
  [in14] -> M146/8(LD)
  M146/1(W1Pos) -> Eval145/1(In1)
  M146/2(W2Pos) -> Eval145/2(In2)
  M146/3(W4Pos) -> Eval145/3(In4)
  Eval145/1(Out1) -> To Workspace145/1
  [in1] -> M147/1(DW1)
  [in4] -> M147/2(DW4)
  [in5] -> M147/3(P1W2)
  [in8] -> M147/4(P3W4)
  [in10] -> M147/5(O1)
  [in11] -> M147/6(O2)
  [in13] -> M147/7(O4)
  [in14] -> M147/8(LD)
  M147/1(W1Pos) -> Eval146/1(In1)
  M147/2(W2Pos) -> Eval146/2(In2)
  M147/3(W4Pos) -> Eval146/3(In4)
  Eval146/1(Out1) -> To Workspace146/1
  [in1] -> M148/1(DW1)
  [in4] -> M148/2(DW4)
  [in5] -> M148/3(P1W2)
  [in8] -> M148/4(P3W4)
  [in10] -> M148/5(O1)
  [in11] -> M148/6(O2)
  [in13] -> M148/7(O4)
  [in14] -> M148/8(LD)
  M148/1(W1Pos) -> Eval147/1(In1)
  M148/2(W2Pos) -> Eval147/2(In2)
  M148/3(W4Pos) -> Eval147/3(In4)
  Eval147/1(Out1) -> To Workspace147/1
  [in1] -> M150/1(DW1)
  [in4] -> M150/2(DW4)
  [in5] -> M150/3(P1W2)
  [in8] -> M150/4(P3W4)
  [in10] -> M150/5(O1)
  [in11] -> M150/6(O2)
  [in13] -> M150/7(O4)
  [in14] -> M150/8(LD)
  M150/1(W1Pos) -> Eval149/1(In1)
  M150/2(W2Pos) -> Eval149/2(In2)
  M150/3(W4Pos) -> Eval149/3(In4)
  Eval149/1(Out1) -> To Workspace149/1
  [in1] -> M151/1(DW1)
  [in4] -> M151/2(DW4)
  [in5] -> M151/3(P1W2)
  [in8] -> M151/4(P3W4)
  [in10] -> M151/5(O1)
  [in11] -> M151/6(O2)
  [in13] -> M151/7(O4)
  [in14] -> M151/8(LD)
  M151/1(W1Pos) -> Eval150/1(In1)
  M151/2(W2Pos) -> Eval150/2(In2)
  M151/3(W4Pos) -> Eval150/3(In4)
  Eval150/1(Out1) -> To Workspace150/1
  [in1] -> M152/1(DW1)
  [in4] -> M152/2(DW4)
  [in5] -> M152/3(P1W2)
  [in8] -> M152/4(P3W4)
  [in10] -> M152/5(O1)
  [in11] -> M152/6(O2)
  [in13] -> M152/7(O4)
  [in14] -> M152/8(LD)
  M152/1(W1Pos) -> Eval151/1(In1)
  M152/2(W2Pos) -> Eval151/2(In2)
  M152/3(W4Pos) -> Eval151/3(In4)
  Eval151/1(Out1) -> To Workspace151/1
  [in1] -> M154/1(DW1)
  [in4] -> M154/2(DW4)
  [in5] -> M154/3(P1W2)
  [in8] -> M154/4(P3W4)
  [in10] -> M154/5(O1)
  [in11] -> M154/6(O2)
  [in13] -> M154/7(O4)
  [in14] -> M154/8(LD)
  M154/1(W1Pos) -> Eval153/1(In1)
  M154/2(W2Pos) -> Eval153/2(In2)
  M154/3(W4Pos) -> Eval153/3(In4)
  Eval153/1(Out1) -> To Workspace153/1
  [in1] -> M155/1(DW1)
  [in4] -> M155/2(DW4)
  [in5] -> M155/3(P1W2)
  [in8] -> M155/4(P3W4)
  [in10] -> M155/5(O1)
  [in11] -> M155/6(O2)
  [in13] -> M155/7(O4)
  [in14] -> M155/8(LD)
  M155/1(W1Pos) -> Eval154/1(In1)
  M155/2(W2Pos) -> Eval154/2(In2)
  M155/3(W4Pos) -> Eval154/3(In4)
  Eval154/1(Out1) -> To Workspace154/1
  [in1] -> M156/1(DW1)
  [in4] -> M156/2(DW4)
  [in5] -> M156/3(P1W2)
  [in8] -> M156/4(P3W4)
  [in10] -> M156/5(O1)
  [in11] -> M156/6(O2)
  [in13] -> M156/7(O4)
  [in14] -> M156/8(LD)
  M156/1(W1Pos) -> Eval155/1(In1)
  M156/2(W2Pos) -> Eval155/2(In2)
  M156/3(W4Pos) -> Eval155/3(In4)
  Eval155/1(Out1) -> To Workspace155/1
  [in1] -> M158/1(DW1)
  [in4] -> M158/2(DW4)
  [in5] -> M158/3(P1W2)
  [in8] -> M158/4(P3W4)
  [in10] -> M158/5(O1)
  [in11] -> M158/6(O2)
  [in13] -> M158/7(O4)
  [in14] -> M158/8(LD)
  M158/1(W1Pos) -> Eval157/1(In1)
  M158/2(W2Pos) -> Eval157/2(In2)
  M158/3(W4Pos) -> Eval157/3(In4)
  Eval157/1(Out1) -> To Workspace157/1
  [in1] -> M159/1(DW1)
  [in4] -> M159/2(DW4)
  [in5] -> M159/3(P1W2)
  [in8] -> M159/4(P3W4)
  [in10] -> M159/5(O1)
  [in11] -> M159/6(O2)
  [in13] -> M159/7(O4)
  [in14] -> M159/8(LD)
  M159/1(W1Pos) -> Eval158/1(In1)
  M159/2(W2Pos) -> Eval158/2(In2)
  M159/3(W4Pos) -> Eval158/3(In4)
  Eval158/1(Out1) -> To Workspace158/1
  [in1] -> M160/1(DW1)
  [in4] -> M160/2(DW4)
  [in5] -> M160/3(P1W2)
  [in8] -> M160/4(P3W4)
  [in10] -> M160/5(O1)
  [in11] -> M160/6(O2)
  [in13] -> M160/7(O4)
  [in14] -> M160/8(LD)
  M160/1(W1Pos) -> Eval159/1(In1)
  M160/2(W2Pos) -> Eval159/2(In2)
  M160/3(W4Pos) -> Eval159/3(In4)
  Eval159/1(Out1) -> To Workspace159/1
  [in1] -> M162/1(DW1)
  [in4] -> M162/2(DW4)
  [in5] -> M162/3(P1W2)
  [in8] -> M162/4(P3W4)
  [in10] -> M162/5(O1)
  [in11] -> M162/6(O2)
  [in13] -> M162/7(O4)
  [in14] -> M162/8(LD)
  M162/1(W1Pos) -> Eval161/1(In1)
  M162/2(W2Pos) -> Eval161/2(In2)
  M162/3(W4Pos) -> Eval161/3(In4)
  Eval161/1(Out1) -> To Workspace161/1
  [in1] -> M163/1(DW1)
  [in4] -> M163/2(DW4)
  [in5] -> M163/3(P1W2)
  [in8] -> M163/4(P3W4)
  [in10] -> M163/5(O1)
  [in11] -> M163/6(O2)
  [in13] -> M163/7(O4)
  [in14] -> M163/8(LD)
  M163/1(W1Pos) -> Eval162/1(In1)
  M163/2(W2Pos) -> Eval162/2(In2)
  M163/3(W4Pos) -> Eval162/3(In4)
  Eval162/1(Out1) -> To Workspace162/1
  [in1] -> M164/1(DW1)
  [in4] -> M164/2(DW4)
  [in5] -> M164/3(P1W2)
  [in8] -> M164/4(P3W4)
  [in10] -> M164/5(O1)
  [in11] -> M164/6(O2)
  [in13] -> M164/7(O4)
  [in14] -> M164/8(LD)
  M164/1(W1Pos) -> Eval163/1(In1)
  M164/2(W2Pos) -> Eval163/2(In2)
  M164/3(W4Pos) -> Eval163/3(In4)
  Eval163/1(Out1) -> To Workspace163/1
  [in1] -> M166/1(DW1)
  [in4] -> M166/2(DW4)
  [in5] -> M166/3(P1W2)
  [in8] -> M166/4(P3W4)
  [in10] -> M166/5(O1)
  [in11] -> M166/6(O2)
  [in13] -> M166/7(O4)
  [in14] -> M166/8(LD)
  M166/1(W1Pos) -> Eval165/1(In1)
  M166/2(W2Pos) -> Eval165/2(In2)
  M166/3(W4Pos) -> Eval165/3(In4)
  Eval165/1(Out1) -> To Workspace165/1
  [in1] -> M167/1(DW1)
  [in4] -> M167/2(DW4)
  [in5] -> M167/3(P1W2)
  [in8] -> M167/4(P3W4)
  [in10] -> M167/5(O1)
  [in11] -> M167/6(O2)
  [in13] -> M167/7(O4)
  [in14] -> M167/8(LD)
  M167/1(W1Pos) -> Eval166/1(In1)
  M167/2(W2Pos) -> Eval166/2(In2)
  M167/3(W4Pos) -> Eval166/3(In4)
  Eval166/1(Out1) -> To Workspace166/1
  [in1] -> M168/1(DW1)
  [in4] -> M168/2(DW4)
  [in5] -> M168/3(P1W2)
  [in8] -> M168/4(P3W4)
  [in10] -> M168/5(O1)
  [in11] -> M168/6(O2)
  [in13] -> M168/7(O4)
  [in14] -> M168/8(LD)
  M168/1(W1Pos) -> Eval167/1(In1)
  M168/2(W2Pos) -> Eval167/2(In2)
  M168/3(W4Pos) -> Eval167/3(In4)
  Eval167/1(Out1) -> To Workspace167/1
  [in1] -> M170/1(DW1)
  [in4] -> M170/2(DW4)
  [in5] -> M170/3(P1W2)
  [in8] -> M170/4(P3W4)
  [in10] -> M170/5(O1)
  [in11] -> M170/6(O2)
  [in13] -> M170/7(O4)
  [in14] -> M170/8(LD)
  M170/1(W1Pos) -> Eval169/1(In1)
  M170/2(W2Pos) -> Eval169/2(In2)
  M170/3(W4Pos) -> Eval169/3(In4)
  Eval169/1(Out1) -> To Workspace169/1
  [in1] -> M171/1(DW1)
  [in4] -> M171/2(DW4)
  [in5] -> M171/3(P1W2)
  [in8] -> M171/4(P3W4)
  [in10] -> M171/5(O1)
  [in11] -> M171/6(O2)
  [in13] -> M171/7(O4)
  [in14] -> M171/8(LD)
  M171/1(W1Pos) -> Eval170/1(In1)
  M171/2(W2Pos) -> Eval170/2(In2)
  M171/3(W4Pos) -> Eval170/3(In4)
  Eval170/1(Out1) -> To Workspace170/1
  [in1] -> M172/1(DW1)
  [in4] -> M172/2(DW4)
  [in5] -> M172/3(P1W2)
  [in8] -> M172/4(P3W4)
  [in10] -> M172/5(O1)
  [in11] -> M172/6(O2)
  [in13] -> M172/7(O4)
  [in14] -> M172/8(LD)
  M172/1(W1Pos) -> Eval171/1(In1)
  M172/2(W2Pos) -> Eval171/2(In2)
  M172/3(W4Pos) -> Eval171/3(In4)
  Eval171/1(Out1) -> To Workspace171/1
  [in1] -> M174/1(DW1)
  [in4] -> M174/2(DW4)
  [in5] -> M174/3(P1W2)
  [in8] -> M174/4(P3W4)
  [in10] -> M174/5(O1)
  [in11] -> M174/6(O2)
  [in13] -> M174/7(O4)
  [in14] -> M174/8(LD)
  M174/1(W1Pos) -> Eval173/1(In1)
  M174/2(W2Pos) -> Eval173/2(In2)
  M174/3(W4Pos) -> Eval173/3(In4)
  Eval173/1(Out1) -> To Workspace173/1
  Inputs/1(DW1) -> dtc_DW1/1
  dtc_DW1/1 -> CPSUT/1(DW1), [in1]
  Inputs/2(DW4) -> dtc_DW4/1
  dtc_DW4/1 -> CPSUT/2(DW4), [in4]
  Inputs/3(P1W2) -> dtc_P1W2/1
  dtc_P1W2/1 -> CPSUT/3(P1W2), [in5]
  Inputs/4(P3W4) -> dtc_P3W4/1
  dtc_P3W4/1 -> CPSUT/4(P3W4), [in8]
  Inputs/5(O1) -> dtc_O1/1
  dtc_O1/1 -> CPSUT/5(O1), [in10]
  Inputs/6(O2) -> dtc_O2/1
  dtc_O2/1 -> CPSUT/6(O2), [in11]
  Inputs/7(O4) -> dtc_O4/1
  dtc_O4/1 -> CPSUT/7(O4), [in13]
  Inputs/8(LD) -> dtc_LD/1
  dtc_LD/1 -> CPSUT/8(LD), [in14]
